simulink model "MBD_Arthimetic1"  (R2021a)
settings: Solver=FixedStepDiscrete  StartTime=0.0  StopTime=100  RelTol=1e-3
libraries: simulink x3
settings Model: Creator=Nour  LastModifiedBy=Nour
settings OptimizationCC: DefaultParameterBehavior=Inlined  EnhancedBackFolding=on  PassReuseOutputArgsAs=Individual arguments  ZeroExternalMemoryAtStartup=off  ZeroInternalMemoryAtStartup=off  OptimizeBlockOrder=speed  DifferentSizesBufferReuse=on  OptimizationCustomize=off  EfficientTunableParamExpr=on
settings DebuggingCC: ParameterTunabilityLossMsg=error
settings SFSimCC: MATLABDynamicMemAlloc=off
settings RTWCC: SystemTargetFile=ert.tlc  GenCodeOnly=on  TemplateMakefile=ert_default_tmf  GenerateReport=on  IncludeHyperlinkInReport=on  LaunchReport=on  GenerateTraceInfo=on
settings CodeAppCC: ForceParamTrailComments=on  IgnoreCustomStorageClasses=off  OperatorAnnotations=on  SimulinkDataObjDesc=on  SFDataObjDesc=on  InsertBlockDesc=on
settings ERTTargetCC: TargetLangStandard=C99 (ISO)  GenerateSampleERTMain=on  InlinedParameterPlacement=NonHierarchical  ERTCustomFileTemplate=example_file_process.tlc

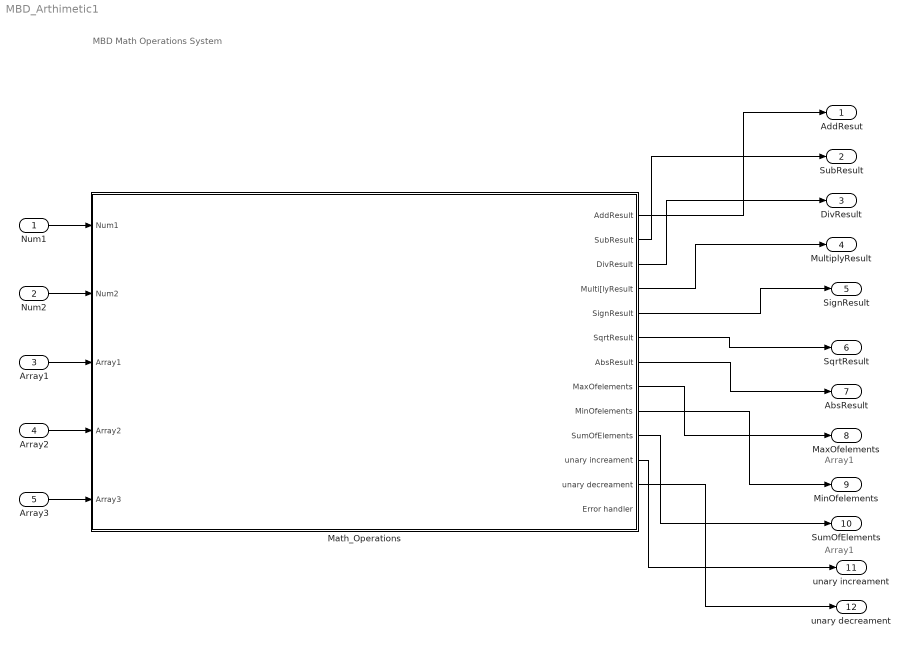
== system MBD_Arthimetic1 ==
  note: MBD Math Operations System
  note: Array1
  note: Array1
  Num1 : Inport
  Num2 : Inport  Port=2
  Array1 : Inport  Port=3
  Array2 : Inport  Port=4
  Array3 : Inport  Port=5
  Math_Operations : Subsystem
  AddResut : Outport
  SubResult : Outport  Port=2
  DivResult : Outport  Port=3
  MultiplyResult : Outport  Port=4
  SignResult : Outport  Port=5
  SqrtResult : Outport  Port=6
  AbsResult : Outport  Port=7
  MaxOfelements : Outport  Port=8
  MinOfelements : Outport  Port=9
  SumOfElements : Outport  Port=10
  unary increament : Outport  Port=11
  unary decreament : Outport  Port=12
  wires:
  Num1/1 -> Math_Operations/1(Num1)
  Num2/1 -> Math_Operations/2(Num2)
  Math_Operations/1(AddResult) -> AddResut/1
  Math_Operations/2(SubResult) -> SubResult/1
  Math_Operations/3(DivResult) -> DivResult/1
  Math_Operations/4(Multi[lyResult) -> MultiplyResult/1
  Math_Operations/5(SignResult) -> SignResult/1
  Math_Operations/6(SqrtResult) -> SqrtResult/1
  Array3/1 -> Math_Operations/5(Array3)
  Array2/1 -> Math_Operations/4(Array2)
  Array1/1 -> Math_Operations/3(Array1)
  Math_Operations/7(AbsResult) -> AbsResult/1
  Math_Operations/8(MaxOfelements) -> MaxOfelements/1
  Math_Operations/10(SumOfElements) -> SumOfElements/1
  Math_Operations/9(MinOfelements) -> MinOfelements/1
  Math_Operations/11(unary increament) -> unary increament/1
  Math_Operations/12(unary decreament) -> unary decreament/1

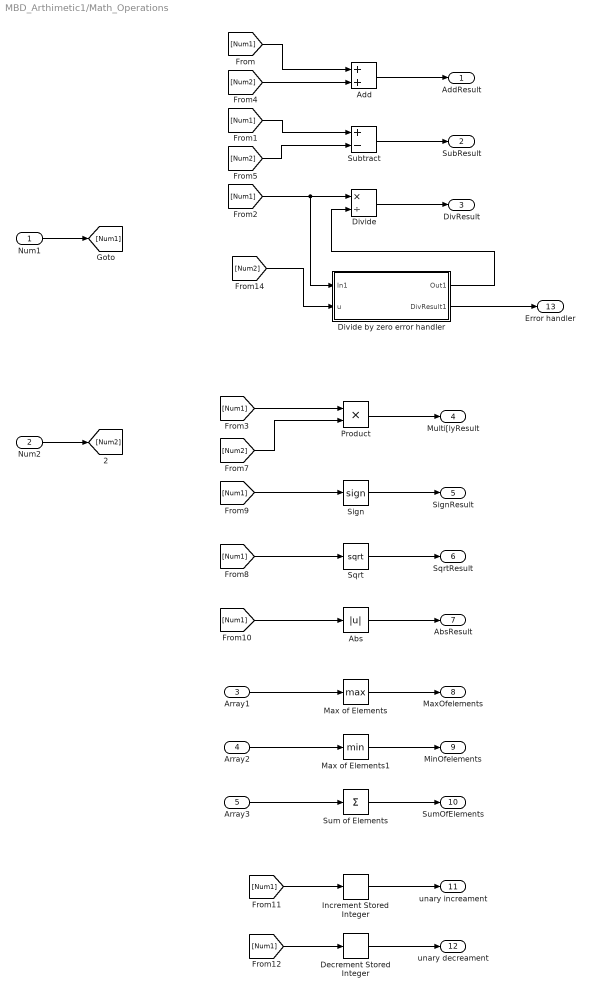
== system MBD_Arthimetic1/Math_Operations ==
  Num1 : Inport  OutDataTypeStr=uint8
  Num2 : Inport  Port=2  OutDataTypeStr=uint8
  Array1 : Inport  Port=3  OutDataTypeStr=uint16  PortDimensions=10
  Array2 : Inport  Port=4  OutDataTypeStr=uint16  PortDimensions=10
  Array3 : Inport  Port=5
  Abs : Abs
  Add : Sum  AccumDataTypeStr=uint8
  Decrement Stored Integer : simulink/Additional Math & Discrete/Additional Math: Increment - Decrement/Decrement Stored Integer
      settings: SourceProductBaseCode=SL
  Divide : Product  Inputs=*/  OutDataTypeStr=uint8
  "Divide by zero error handler " : Subsystem
  Increment Stored Integer : simulink/Additional Math & Discrete/Additional Math: Increment - Decrement/Increment Stored Integer
  Max of Elements : MinMax  Function=max
  Max of Elements1 : MinMax  OutDataTypeStr=uint16
  Product : Product  OutDataTypeStr=uint8
  Sign : Signum
  Sqrt : Sqrt  SaturateOnIntegerOverflow=on
  Subtract : Sum  Inputs=+-  AccumDataTypeStr=int8
  Sum of Elements : Sum  Inputs=+  AccumDataTypeStr=uint16
  AddResult : Outport
  SubResult : Outport  Port=2
  DivResult : Outport  Port=3
  Multi[lyResult : Outport  Port=4
  SignResult : Outport  Port=5
  SqrtResult : Outport  Port=6
  AbsResult : Outport  Port=7
  MaxOfelements : Outport  Port=8
  MinOfelements : Outport  Port=9
  SumOfElements : Outport  Port=10
  unary increament : Outport  Port=11
  unary decreament : Outport  Port=12
  Error handler : Outport  Port=13
  wires:
  Subtract/1 -> SubResult/1
  Add/1 -> AddResult/1
  Product/1 -> Multi[lyResult/1
  Divide/1 -> DivResult/1
  Num1/1 -> [Num1]
  Num2/1 -> [Num2]
  [Num1] -> Add/1
  [Num1] -> Subtract/1
  [Num1] -> Product/1
  [Num2] -> Add/2
  [Num2] -> Subtract/2
  [Num2] -> Product/2
  [Num1] -> Sign/1
  [Num1] -> Sqrt/1
  Sign/1 -> SignResult/1
  Sqrt/1 -> SqrtResult/1
  [Num1] -> Abs/1
  Abs/1 -> AbsResult/1
  Array1/1 -> Max of Elements/1
  Array3/1 -> Sum of Elements/1
  Array2/1 -> Max of Elements1/1
  Max of Elements/1 -> MaxOfelements/1
  Sum of Elements/1 -> SumOfElements/1
  Max of Elements1/1 -> MinOfelements/1
  [Num1] -> Increment Stored Integer/1
  [Num1] -> Decrement Stored Integer/1
  Increment Stored Integer/1 -> unary increament/1
  Decrement Stored Integer/1 -> unary decreament/1
  [Num1] -> "Divide by zero error handler "/1(In1), Divide/1
  [Num2] -> "Divide by zero error handler "/2(u)
  "Divide by zero error handler "/1(Out1) -> Divide/2
  "Divide by zero error handler "/2(DivResult1) -> Error handler/1

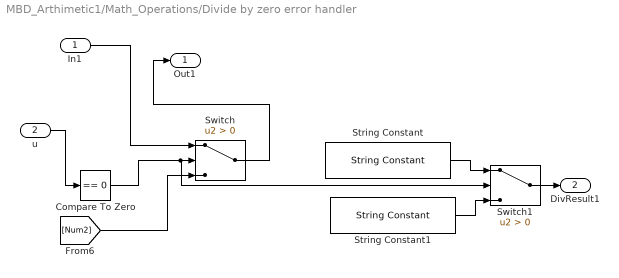
== system MBD_Arthimetic1/Math_Operations/Divide by zero error handler  ==
  In1 : Inport
  u : Inport  Port=2
  Compare To Zero : simulink/Logic and Bit Operations/Compare To Zero  relop===  OutDataTypeStr=boolean
  String Constant : StringConstant  String="\"Error!!! can't Divide by zero\""
  String Constant1 : StringConstant  String="\"operation Done\""
  Switch : Switch  Criteria=u2 > Threshold
  Switch1 : Switch  Criteria=u2 > Threshold
  Out1 : Outport
  DivResult1 : Outport  Port=2
  wires:
  Switch1/1 -> DivResult1/1
  Compare To Zero/1 -> Switch1/2, Switch/2
  String Constant1/1 -> Switch1/3
  [Num2] -> Switch/3
  String Constant/1 -> Switch1/1
  Switch/1 -> Out1/1
  In1/1 -> Switch/1
  u/1 -> Compare To Zero/1
